simulink model "Kettle_System"  (R2018b)
settings: Solver=FixedStepAuto  StartTime=0.0  StopTime=500  FixedStep=1  RelTol=1e-3
settings Model: DataTypeOverride=Double  MinMaxOverflowLogging=ForceOff  Creator=georgimarkov  LastModifiedBy=r1pp3r
settings SFSimCC: SimUseLocalCustomCode=off
settings RTWCC: RTWUseLocalCustomCode=off

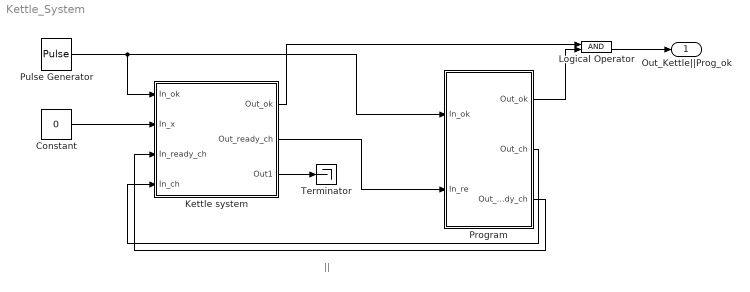
== system Kettle_System ==
  note: ||
  Constant : Constant  Value=0
  "Kettle system " : Subsystem
  Logical Operator : Logic  AllPortsSameDT=off  OutDataTypeStr=boolean
  Program : Subsystem
  Pulse Generator : DiscretePulseGenerator  Period=5  PulseWidth=3  PhaseDelay=1  SampleTime=30
  Terminator : Terminator
  Out_Kettle||Prog_ok : Outport
  wires:
  Pulse Generator/1 -> "Kettle system "/1(In_ok), Program/1(In_ok)
  "Kettle system "/2(Out_ready_ch) -> Program/2(In_re)
  Program/1(Out_ok) -> Logical Operator/2
  "Kettle system "/1(Out_ok) -> Logical Operator/1
  Logical Operator/1 -> Out_Kettle||Prog_ok/1
  Program/3("Out_ready_ch ") -> "Kettle system "/3(In_ready_ch)
  Program/2(Out_ch) -> "Kettle system "/4(In_ch)
  Constant/1 -> "Kettle system "/2(In_x)
  "Kettle system "/3(Out1) -> Terminator/1

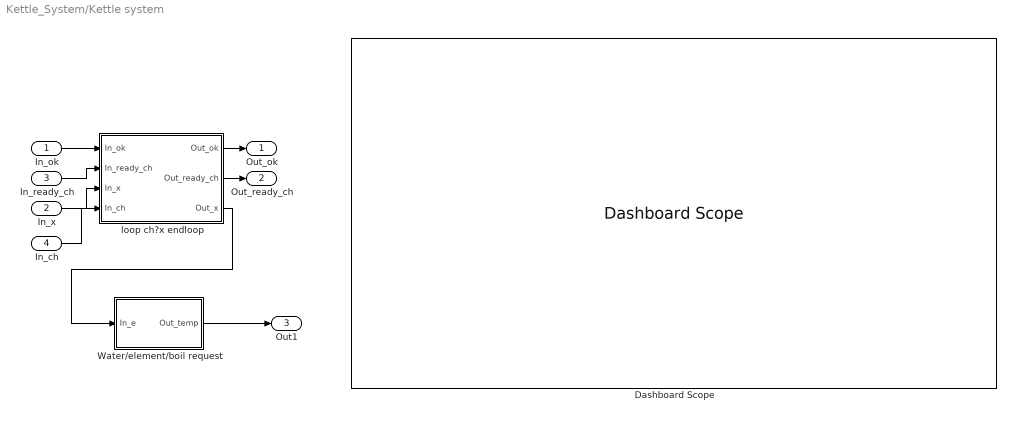
== system Kettle_System/Kettle system  ==
  In_ok : Inport
  In_x : Inport  Port=2
  In_ready_ch : Inport  Port=3
  In_ch : Inport  Port=4
  Dashboard Scope : DashboardScope  WebBlockId=661  Ymin=10  Ymax=110
  Water/element/boil request : Subsystem
  loop ch?x endloop : Subsystem
  Out_ok : Outport
  Out_ready_ch : Outport  Port=2
  Out1 : Outport  Port=3
  wires:
  Water/element/boil request/1(Out_temp) -> Out1/1
  In_ok/1 -> loop ch?x endloop/1(In_ok)
  In_x/1 -> loop ch?x endloop/3(In_x)
  loop ch?x endloop/1(Out_ok) -> Out_ok/1
  loop ch?x endloop/3(Out_x) -> Water/element/boil request/1(In_e)
  In_ready_ch/1 -> loop ch?x endloop/2(In_ready_ch)
  loop ch?x endloop/2(Out_ready_ch) -> Out_ready_ch/1
  In_ch/1 -> loop ch?x endloop/4(In_ch)

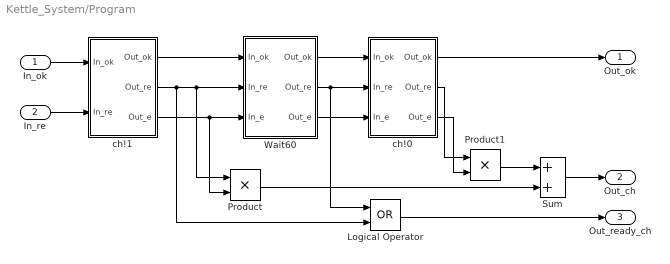
== system Kettle_System/Program ==
  In_ok : Inport
  In_re : Inport  Port=2
  Logical Operator : Logic  Operator=OR  AllPortsSameDT=off  OutDataTypeStr=fixdt(1,16)
  Product : Product
  Product1 : Product
  Sum : Sum
  Wait60 : Subsystem
  ch!0 : Subsystem
  "ch!1 " : Subsystem
  Out_ok : Outport
  Out_ch : Outport  Port=2
  "Out_ready_ch " : Outport  Port=3
  wires:
  "ch!1 "/2(Out_re) -> Product/1, Wait60/2(In_re), Logical Operator/2
  In_ok/1 -> "ch!1 "/1(In_ok)
  Wait60/2(Out_re) -> ch!0/2(In_re), Logical Operator/1
  Wait60/1(Out_ok) -> ch!0/1(In_ok)
  ch!0/1(Out_ok) -> Out_ok/1
  ch!0/3(Out_e) -> Product1/2
  "ch!1 "/1(Out_ok) -> Wait60/1("In_ok ")
  "ch!1 "/3(Out_e) -> Product/2, Wait60/3(In_e)
  In_re/1 -> "ch!1 "/2(In_re)
  ch!0/2(Out_re) -> Product1/1
  Sum/1 -> Out_ch/1
  Logical Operator/1 -> "Out_ready_ch "/1
  Wait60/3(Out_e) -> ch!0/3("In_e ")
  Product1/1 -> Sum/1
  Product/1 -> Sum/2

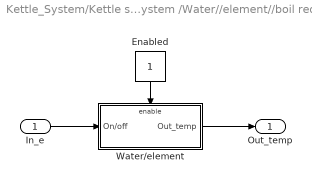
== system Kettle_System/Kettle system /Water//element//boil request ==
  In_e : Inport
  Enabled : Constant
  Water/element : Subsystem  TreatAsAtomicUnit=on
  Out_temp : Outport
  wires:
  Water/element/1("Out_temp ") -> Out_temp/1
  In_e/1 -> Water/element/1(On/off)
  Enabled/1 -> Water/element/Enable

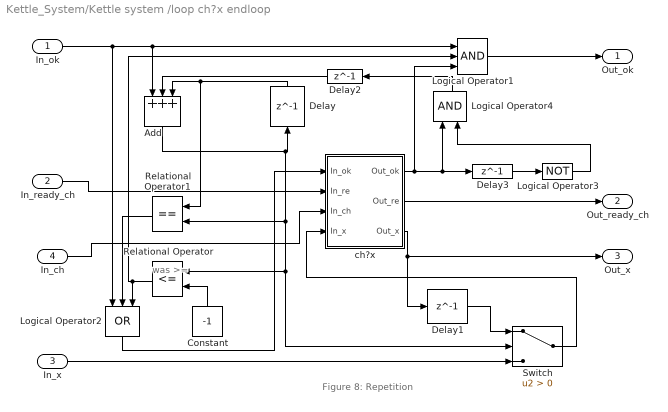
== system Kettle_System/Kettle system /loop ch?x endloop ==
  note: was >=
  note: Figure 8: Repetition
  In_ok : Inport
  In_ready_ch : Inport  Port=2
  In_x : Inport  Port=3
  In_ch : Inport  Port=4
  Add : Sum  Inputs=+++
  Constant : Constant  Value=-1
  Delay{,1..3} (4 alike) : Delay  DelayLength=1  InitialCondition=0
  Logical Operator1 : Logic  Inputs=3  AllPortsSameDT=off  OutDataTypeStr=fixdt(1,16)
  Logical Operator2 : Logic  Operator=OR  Inputs=3  AllPortsSameDT=off  OutDataTypeStr=fixdt(1,16)
  Logical Operator3 : Logic  Operator=NOT  AllPortsSameDT=off  OutDataTypeStr=fixdt(1,16)
  Logical Operator4 : Logic  AllPortsSameDT=off  OutDataTypeStr=fixdt(1,16)
  Relational Operator : RelationalOperator  Operator=<=  OutDataTypeStr=boolean  RndMeth=Simplest
  Relational Operator1 : RelationalOperator  Operator===  OutDataTypeStr=boolean  RndMeth=Simplest
  Switch : Switch  Criteria=u2 > Threshold  OutDataTypeStr=double
  ch?x : Subsystem
  Out_ok : Outport
  Out_ready_ch : Outport  Port=2
  Out_x : Outport  Port=3
  wires:
  In_ok/1 -> Add/1, Logical Operator1/1, Logical Operator2/1
  Logical Operator1/1 -> Out_ok/1
  In_x/1 -> Switch/3
  ch?x/3("Out_x ") -> Delay1/1, Out_x/1
  Logical Operator4/1 -> Delay2/1
  Delay1/1 -> Switch/1
  Relational Operator/1 -> Logical Operator1/2, Logical Operator2/3
  ch?x/1(Out_ok) -> Delay3/1, Logical Operator4/1, Logical Operator1/3
  Logical Operator2/1 -> ch?x/1(In_ok)
  Delay3/1 -> Logical Operator3/1
  Constant/1 -> Relational Operator/2
  Add/1 -> Relational Operator1/2, Switch/2, Relational Operator/1, Delay/1
  ch?x/2(Out_re) -> Out_ready_ch/1
  Delay2/1 -> Add/2
  Relational Operator1/1 -> Logical Operator2/2
  Logical Operator3/1 -> Logical Operator4/2
  Delay/1 -> Add/3, Relational Operator1/1
  In_ready_ch/1 -> ch?x/2(In_re)
  In_ch/1 -> ch?x/3(In_ch)
  Switch/1 -> ch?x/4(In_x)

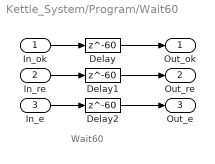
== system Kettle_System/Program/Wait60 ==
  note: Wait60
  "In_ok " : Inport
  In_re : Inport  Port=2
  In_e : Inport  Port=3
  Delay : Delay  DelayLength=60  InitialCondition=0
  Delay1 : Delay  DelayLength=60  InitialCondition=0
  Delay2 : Delay  DelayLength=60  InitialCondition=0
  Out_ok : Outport
  Out_re : Outport  Port=2
  Out_e : Outport  Port=3
  wires:
  Delay1/1 -> Out_re/1
  In_e/1 -> Delay2/1
  In_re/1 -> Delay1/1
  Delay2/1 -> Out_e/1
  Delay/1 -> Out_ok/1
  "In_ok "/1 -> Delay/1

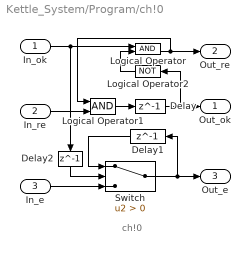
== system Kettle_System/Program/ch!0 ==
  note: ch!0
  In_ok : Inport
  In_re : Inport  Port=2
  "In_e " : Inport  Port=3
  Delay : Delay  DelayLength=1  InitialCondition=0
  Delay1 : Delay  DelayLength=1  InitialCondition=0
  Delay2 : Delay  DelayLength=1  InitialCondition=0
  Logical Operator : Logic  AllPortsSameDT=off  OutDataTypeStr=fixdt(1,16)
  Logical Operator1 : Logic  AllPortsSameDT=off  OutDataTypeStr=fixdt(1,16)
  Logical Operator2 : Logic  Operator=NOT  AllPortsSameDT=off  OutDataTypeStr=fixdt(1,16)
  Switch : Switch  Criteria=u2 > Threshold
  Out_ok : Outport
  Out_re : Outport  Port=2
  Out_e : Outport  Port=3
  wires:
  In_re/1 -> Logical Operator1/2
  Logical Operator2/1 -> Logical Operator/2
  Logical Operator1/1 -> Delay/1
  In_ok/1 -> Logical Operator/1, Delay2/1
  Delay2/1 -> Switch/2
  Logical Operator/1 -> Out_re/1, Logical Operator1/1
  Switch/1 -> Delay1/1, Out_e/1
  Delay1/1 -> Switch/1
  "In_e "/1 -> Switch/3
  Delay/1 -> Out_ok/1, Logical Operator2/1

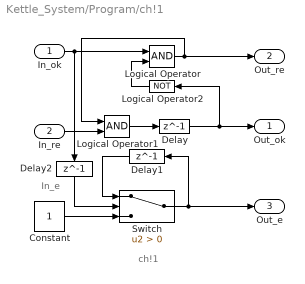
== system Kettle_System/Program/ch!1  ==
  note: In_e
  note: ch!1
  In_ok : Inport
  In_re : Inport  Port=2
  Constant : Constant
  Delay : Delay  DelayLength=1  InitialCondition=0
  Delay1 : Delay  DelayLength=1  InitialCondition=0
  Delay2 : Delay  DelayLength=1  InitialCondition=0
  Logical Operator : Logic  AllPortsSameDT=off  OutDataTypeStr=fixdt(1,16)
  Logical Operator1 : Logic  AllPortsSameDT=off  OutDataTypeStr=fixdt(1,16)
  Logical Operator2 : Logic  Operator=NOT  AllPortsSameDT=off  OutDataTypeStr=boolean
  Switch : Switch  Criteria=u2 > Threshold
  Out_ok : Outport
  Out_re : Outport  Port=2
  Out_e : Outport  Port=3
  wires:
  In_re/1 -> Logical Operator1/2
  Logical Operator2/1 -> Logical Operator/2
  In_ok/1 -> Delay2/1, Logical Operator/1
  Delay2/1 -> Switch/2
  Switch/1 -> Delay1/1, Out_e/1
  Delay1/1 -> Switch/1
  Constant/1 -> Switch/3
  Logical Operator/1 -> Out_re/1, Logical Operator1/1
  Logical Operator1/1 -> Delay/1
  Delay/1 -> Logical Operator2/1, Out_ok/1

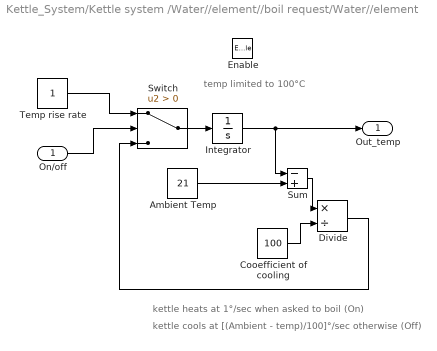
== system Kettle_System/Kettle system /Water//element//boil request/Water//element ==
  note: temp limited to 100°C
  note: kettle heats at 1°/sec when asked to boil (On)
  note: kettle cools at [(Ambient - temp)/100]°/sec otherwise (Off)
  On/off : Inport
  Enable : EnablePort
  "Ambient Temp " : Constant  Value=21
  Cooefficient of cooling : Constant  Value=100
  Divide : Product  Inputs=*/
  Integrator : Integrator  InitialCondition=21  LimitOutput=on  UpperSaturationLimit=100  ContinuousStateAttributes='temp'
  Sum : Sum  Inputs=-+
  Switch : Switch  Criteria=u2 > Threshold
  Temp rise rate : Constant
  "Out_temp " : Outport
  wires:
  On/off/1 -> Switch/2
  Integrator/1 -> Sum/1, "Out_temp "/1
  Switch/1 -> Integrator/1
  Temp rise rate/1 -> Switch/1
  "Ambient Temp "/1 -> Sum/2
  Sum/1 -> Divide/1
  Cooefficient of cooling/1 -> Divide/2
  Divide/1 -> Switch/3

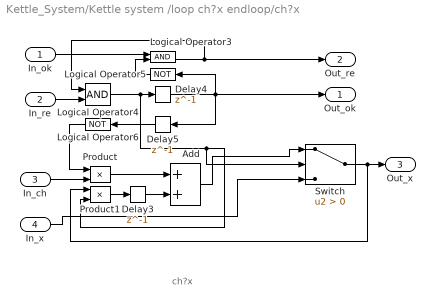
== system Kettle_System/Kettle system /loop ch?x endloop/ch?x ==
  note: ch?x
  In_ok : Inport
  In_re : Inport  Port=2
  In_ch : Inport  Port=3
  In_x : Inport  Port=4
  Add : Sum
  Delay3 : Delay  DelayLength=1  InitialCondition=0
  Delay4 : Delay  DelayLength=1  InitialCondition=0
  Delay5 : Delay  DelayLength=1  InitialCondition=0
  Logical Operator3 : Logic  AllPortsSameDT=off  OutDataTypeStr=fixdt(1,16)
  Logical Operator4 : Logic  AllPortsSameDT=off  OutDataTypeStr=fixdt(1,16)
  Logical Operator5 : Logic  Operator=NOT  AllPortsSameDT=off  OutDataTypeStr=fixdt(1,16)
  Logical Operator6 : Logic  Operator=NOT  AllPortsSameDT=off  OutDataTypeStr=fixdt(1,16)
  Product : Product
  Product1 : Product
  Switch : Switch  Criteria=u2 > Threshold
  Out_ok : Outport
  Out_re : Outport  Port=2
  "Out_x " : Outport  Port=3
  wires:
  In_ch/1 -> Product/2
  In_ok/1 -> Logical Operator3/1
  Delay4/1 -> Delay5/1, Logical Operator5/1, Out_ok/1
  Product1/1 -> Delay3/1
  Logical Operator4/1 -> Product1/2, Switch/2, Delay4/1
  In_re/1 -> Logical Operator4/2
  Logical Operator5/1 -> Logical Operator3/2
  Product/1 -> Add/1
  Delay3/1 -> Add/2
  Logical Operator6/1 -> Product/1
  Add/1 -> Switch/1
  Delay5/1 -> Logical Operator6/1
  Logical Operator3/1 -> Out_re/1, Logical Operator4/1
  In_x/1 -> Switch/3
  Switch/1 -> Product1/1, "Out_x "/1
